simulink model "vardownsampler"  (Simulink 7.3)
settings: Solver=VariableStepDiscrete  StartTime=0.0  StopTime=simTime*SampleTime  RelTol=1e-3
PreLoadFcn:
  | setup_vardownsampler
InitFcn:
  | setup_vardownsampler
values from neighbouring files (symbols this model uses):
  accumOutShift = [1 4 3 2 4]    [setup_vardownsampler.m]    (also in setup_vardownsamplerL8.m = [3 3 2 2 2])
  accumOutWidth = dataWidth + ceil(log2(Rmax))+0    [setup_vardownsampler.m]    (also in setup_vardownsamplerL8.m)
  adderOutShift = 4*ones(1,numRates)    [setup_vardownsampler.m]    (also in setup_vardownsamplerL8.m = 3*ones(1,numRates))
  adderOutWidth = dataWidth + coeffWidth + ceil(log2(L))    [setup_vardownsampler.m]    (also in setup_vardownsamplerL8.m)
  addrWidth = max(1,ceil(log2(Rmax)))    [setup_vardownsampler.m]    (also in setup_vardownsamplerL8.m)
  ChanCount = 16    [setup_vardownsampler.m]    (also in setup_vardownsamplerL8.m = 1)
  ChanCycleCount = ceil(ChanCount/ChanWireCount)    [setup_vardownsampler.m]    (also in setup_vardownsamplerL8.m)
  ChanWireCount = ceil(ChanCount/Period)    [setup_vardownsampler.m]    (also in setup_vardownsamplerL8.m)
  coeffWidth = 16    [setup_vardownsampler.m]    (also in setup_vardownsamplerL8.m)
  dataWidth = 16    [setup_vardownsampler.m]    (also in setup_vardownsamplerL8.m)
  FirAddr = AccumOutScale + 1    (= 4)    [setup_vardownsampler.m]    (also in setup_vardownsamplerL8.m)
  hmatrix = zeros(2*Rmax, L)    [setup_vardownsampler.m]    (also in setup_vardownsamplerL8.m)
  memAddrWidth = max(1,ceil(log2(Nmax)))    [setup_vardownsampler.m]    (also in setup_vardownsamplerL8.m)
  Nmax = Period*Rmax    [setup_vardownsampler.m]    (also in setup_vardownsamplerL8.m)
  Period = floor(ClockRate / SampleRate)    [setup_vardownsampler.m]    (also in setup_vardownsamplerL8.m)
  R = [1 2 5 8 2]    [setup_vardownsampler.m]    (also in setup_vardownsamplerL8.m = [4 5 7 8 9])
  RateWidth = ceil(log2(Rmax))+1    [setup_vardownsampler.m]    (also in setup_vardownsamplerL8.m)
  resetCntWidth = max(1,ceil(log2(Nmax)))    [setup_vardownsampler.m]    (also in setup_vardownsamplerL8.m)
  Rmax = 16    [setup_vardownsampler.m]    (also in setup_vardownsamplerL8.m = 20)
  SampleTime = 1    [setup_vardownsampler.m]    (also in setup_vardownsamplerL8.m)
undefined symbols (not defined in the file or in its folder): AdvDSPBChannelOutDisplay, AdvDSPBDMemDisplay, bank1, bank2, c4, c5, c6, c7, c8, c9, dpoly, dspba_ChannelInVis, dspba_ChannelOutVis, dspba_internal_get_channel_ports, evalAionMaskParam, hmatrix0, hmatrix1, hmatrix2, hmatrix3, latency, primtype, UseDontCare, value
libraries: DSPBAPrim x314, DSPBAModelBus x24, simulink x12, DSPBABase x6
(part 4 of 4)

== system vardownsampler/FilterSystem/coefficients_gen/c2 ==
  addr : Inport
  offset : Inport  Port=2
  Const : DSPBAPrim/Const  primtype=const  nInputs=0  nOutputs=1  omode=Specify via dialog  otype=sfix(coeffWidth)  scale=2^-15  rndmethod=Unbiased  factor=1  satmethod=Symmetric  shift_vec=[0 1 2 -1]  value=0  inPortNames=['+'; '+';]  outPortNames=[' ']  image=dspba_prim.jpg  text=fprintf('%s', num2str(value));  style=Optimised  visibilities=8 + 1024  version=20090407
  Const1 : DSPBAPrim/Const  primtype=const  nInputs=0  nOutputs=1  omode=boolean  otype=sfix(16)  scale=2^-15  rndmethod=Unbiased  factor=1  satmethod=Symmetric  shift_vec=[0 1 2 -1]  value=0  inPortNames=['+'; '+';]  outPortNames=[' ']  image=dspba_prim.jpg  text=fprintf('%s', num2str(value));  style=Optimised  visibilities=8 + 1024  version=20090407
  Const2 : DSPBAPrim/Const  primtype=const  nInputs=0  nOutputs=1  omode=Specify via dialog  otype=sfix(coeffWidth)  scale=2^-15  rndmethod=Unbiased  factor=1  satmethod=Symmetric  shift_vec=[0 1 2 -1]  value=0  inPortNames=['+'; '+';]  outPortNames=[' ']  image=dspba_prim.jpg  text=fprintf('%s', num2str(value));  style=Optimised  visibilities=8 + 1024  version=20090407
  Const3 : DSPBAPrim/Const  primtype=const  nInputs=0  nOutputs=1  omode=boolean  otype=sfix(16)  scale=2^-15  rndmethod=Unbiased  factor=1  satmethod=Symmetric  shift_vec=[0 1 2 -1]  value=0  inPortNames=['+'; '+';]  outPortNames=[' ']  image=dspba_prim.jpg  text=fprintf('%s', num2str(value));  style=Optimised  visibilities=8 + 1024  version=20090407
  LUT0 : DSPBAModelBus/SharedMem  mem_addr=FirAddr+ 4*Rmax  mem_rwmode=Read/Write  mem_data=hmatrix(1:Rmax,3)  mem_init=on  mem_desc=hmatrix2-bank1  mem_type=sfix(coeffWidth)  mem_scale=2^-(coeffWidth-1)  SampleTime=-1  version=20090407
  LUT1 : DSPBAModelBus/SharedMem  mem_addr=FirAddr+ 5*Rmax  mem_rwmode=Read/Write  mem_data=hmatrix(Rmax+1:2*Rmax,3)  mem_init=on  mem_desc=hmatrix2-bank2  mem_type=sfix(coeffWidth)  mem_scale=2^-(coeffWidth-1)  SampleTime=-1  version=20090407
  Mux : DSPBAPrim/Mux  primtype=mux  nInputs=evalAionMaskParam(gcb,'value',1)+1  nOutputs=1  omode=Inherit via internal rule  otype=sfix(16)  scale=2^-15  rndmethod=Unbiased  factor=1  satmethod=Symmetric  shift_vec=[0 1 2 -1]  value=2  inPortNames=['s'; 'd0'; 'd1'; 'd2'; 'd3'; 'd4'; 'd5'; 'd6'; 'd7'; 'd8'; 'd9';]  outPortNames=[' ']  image=dspba_prim.jpg  text=fprintf('%s', primtype);  style=Optimised  visibilities=1032  version=20090623
  Out1 : Outport
  wires:
  addr/1 -> LUT0/1, LUT1/1
  Const2/1 -> LUT1/2
  Const3/1 -> LUT1/3
  Const/1 -> LUT0/2
  Const1/1 -> LUT0/3
  Mux/1 -> Out1/1
  offset/1 -> Mux/1
  LUT0/1 -> Mux/2
  LUT1/1 -> Mux/3

== system vardownsampler/FilterSystem/coefficients_gen/c3 ==
  addr : Inport
  offset : Inport  Port=2
  Const : DSPBAPrim/Const  primtype=const  nInputs=0  nOutputs=1  omode=Specify via dialog  otype=sfix(coeffWidth)  scale=2^-15  rndmethod=Unbiased  factor=1  satmethod=Symmetric  shift_vec=[0 1 2 -1]  value=0  inPortNames=['+'; '+';]  outPortNames=[' ']  image=dspba_prim.jpg  text=fprintf('%s', num2str(value));  style=Optimised  visibilities=8 + 1024  version=20090407
  Const1 : DSPBAPrim/Const  primtype=const  nInputs=0  nOutputs=1  omode=boolean  otype=sfix(16)  scale=2^-15  rndmethod=Unbiased  factor=1  satmethod=Symmetric  shift_vec=[0 1 2 -1]  value=0  inPortNames=['+'; '+';]  outPortNames=[' ']  image=dspba_prim.jpg  text=fprintf('%s', num2str(value));  style=Optimised  visibilities=8 + 1024  version=20090407
  Const2 : DSPBAPrim/Const  primtype=const  nInputs=0  nOutputs=1  omode=Specify via dialog  otype=sfix(coeffWidth)  scale=2^-15  rndmethod=Unbiased  factor=1  satmethod=Symmetric  shift_vec=[0 1 2 -1]  value=0  inPortNames=['+'; '+';]  outPortNames=[' ']  image=dspba_prim.jpg  text=fprintf('%s', num2str(value));  style=Optimised  visibilities=8 + 1024  version=20090407
  Const3 : DSPBAPrim/Const  primtype=const  nInputs=0  nOutputs=1  omode=boolean  otype=sfix(16)  scale=2^-15  rndmethod=Unbiased  factor=1  satmethod=Symmetric  shift_vec=[0 1 2 -1]  value=0  inPortNames=['+'; '+';]  outPortNames=[' ']  image=dspba_prim.jpg  text=fprintf('%s', num2str(value));  style=Optimised  visibilities=8 + 1024  version=20090407
  LUT1 : DSPBAModelBus/SharedMem  mem_addr=FirAddr+ 7*Rmax  mem_rwmode=Read/Write  mem_data=hmatrix(Rmax+1:2*Rmax,4)  mem_init=on  mem_desc=hmatrix3-bank2  mem_type=sfix(coeffWidth)  mem_scale=2^-(coeffWidth-1)  SampleTime=-1  version=20090407
  LUT3 : DSPBAModelBus/SharedMem  mem_addr=FirAddr+ 6*Rmax  mem_rwmode=Read/Write  mem_data=hmatrix(1:Rmax,4)  mem_init=on  mem_desc=hmatrix3-bank1  mem_type=sfix(coeffWidth)  mem_scale=2^-(coeffWidth-1)  SampleTime=-1  version=20090407
  Mux : DSPBAPrim/Mux  primtype=mux  nInputs=evalAionMaskParam(gcb,'value',1)+1  nOutputs=1  omode=Inherit via internal rule  otype=sfix(16)  scale=2^-15  rndmethod=Unbiased  factor=1  satmethod=Symmetric  shift_vec=[0 1 2 -1]  value=2  inPortNames=['s'; 'd0'; 'd1'; 'd2'; 'd3'; 'd4'; 'd5'; 'd6'; 'd7'; 'd8'; 'd9';]  outPortNames=[' ']  image=dspba_prim.jpg  text=fprintf('%s', primtype);  style=Optimised  visibilities=1032  version=20090623
  c3 : Outport
  wires:
  addr/1 -> LUT3/1, LUT1/1
  Const/1 -> LUT3/2
  Const1/1 -> LUT3/3
  Const2/1 -> LUT1/2
  Const3/1 -> LUT1/3
  offset/1 -> Mux/1
  LUT3/1 -> Mux/2
  LUT1/1 -> Mux/3
  Mux/1 -> c3/1

== system vardownsampler/FilterSystem/coefficients_gen/c4 ==
  addr : Inport
  offset : Inport  Port=2
  Const : DSPBAPrim/Const  primtype=const  nInputs=0  nOutputs=1  omode=Specify via dialog  otype=sfix(coeffWidth)  scale=2^-15  rndmethod=Unbiased  factor=1  satmethod=Symmetric  shift_vec=[0 1 2 -1]  value=0  inPortNames=['+'; '+';]  outPortNames=[' ']  image=dspba_prim.jpg  text=fprintf('%s', num2str(value));  style=Optimised  visibilities=8 + 1024  version=20090407
  Const1 : DSPBAPrim/Const  primtype=const  nInputs=0  nOutputs=1  omode=boolean  otype=sfix(16)  scale=2^-15  rndmethod=Unbiased  factor=1  satmethod=Symmetric  shift_vec=[0 1 2 -1]  value=0  inPortNames=['+'; '+';]  outPortNames=[' ']  image=dspba_prim.jpg  text=fprintf('%s', num2str(value));  style=Optimised  visibilities=8 + 1024  version=20090407
  Const2 : DSPBAPrim/Const  primtype=const  nInputs=0  nOutputs=1  omode=Specify via dialog  otype=sfix(coeffWidth)  scale=2^-15  rndmethod=Unbiased  factor=1  satmethod=Symmetric  shift_vec=[0 1 2 -1]  value=0  inPortNames=['+'; '+';]  outPortNames=[' ']  image=dspba_prim.jpg  text=fprintf('%s', num2str(value));  style=Optimised  visibilities=8 + 1024  version=20090407
  Const3 : DSPBAPrim/Const  primtype=const  nInputs=0  nOutputs=1  omode=boolean  otype=sfix(16)  scale=2^-15  rndmethod=Unbiased  factor=1  satmethod=Symmetric  shift_vec=[0 1 2 -1]  value=0  inPortNames=['+'; '+';]  outPortNames=[' ']  image=dspba_prim.jpg  text=fprintf('%s', num2str(value));  style=Optimised  visibilities=8 + 1024  version=20090407
  LUT0 : DSPBAModelBus/SharedMem  mem_addr=FirAddr+8*Rmax  mem_rwmode=Read/Write  mem_data=hmatrix(1:Rmax,5)  mem_init=on  mem_desc=c4-bank1  mem_type=sfix(coeffWidth)  mem_scale=2^-(coeffWidth-1)  SampleTime=-1  version=20090407
  LUT1 : DSPBAModelBus/SharedMem  mem_addr=FirAddr+9*Rmax  mem_rwmode=Read/Write  mem_data=hmatrix(Rmax+1:2*Rmax,5)  mem_init=on  mem_desc=c4-bank2  mem_type=sfix(coeffWidth)  mem_scale=2^-(coeffWidth-1)  SampleTime=-1  version=20090407
  Mux : DSPBAPrim/Mux  primtype=mux  nInputs=evalAionMaskParam(gcb,'value',1)+1  nOutputs=1  omode=Inherit via internal rule  otype=sfix(16)  scale=2^-15  rndmethod=Unbiased  factor=1  satmethod=Symmetric  shift_vec=[0 1 2 -1]  value=2  inPortNames=['s'; 'd0'; 'd1'; 'd2'; 'd3'; 'd4'; 'd5'; 'd6'; 'd7'; 'd8'; 'd9';]  outPortNames=[' ']  image=dspba_prim.jpg  text=fprintf('%s', primtype);  style=Optimised  visibilities=1032  version=20090623
  c4 : Outport
  wires:
  addr/1 -> LUT0/1, LUT1/1
  Const/1 -> LUT0/2
  Const1/1 -> LUT0/3
  Const2/1 -> LUT1/2
  Const3/1 -> LUT1/3
  offset/1 -> Mux/1
  LUT0/1 -> Mux/2
  LUT1/1 -> Mux/3
  Mux/1 -> c4/1

== system vardownsampler/FilterSystem/coefficients_gen/c5 ==
  addr : Inport
  offset : Inport  Port=2
  Const : DSPBAPrim/Const  primtype=const  nInputs=0  nOutputs=1  omode=Specify via dialog  otype=sfix(coeffWidth)  scale=2^-15  rndmethod=Unbiased  factor=1  satmethod=Symmetric  shift_vec=[0 1 2 -1]  value=0  inPortNames=['+'; '+';]  outPortNames=[' ']  image=dspba_prim.jpg  text=fprintf('%s', num2str(value));  style=Optimised  visibilities=8 + 1024  version=20090407
  Const1 : DSPBAPrim/Const  primtype=const  nInputs=0  nOutputs=1  omode=boolean  otype=sfix(16)  scale=2^-15  rndmethod=Unbiased  factor=1  satmethod=Symmetric  shift_vec=[0 1 2 -1]  value=0  inPortNames=['+'; '+';]  outPortNames=[' ']  image=dspba_prim.jpg  text=fprintf('%s', num2str(value));  style=Optimised  visibilities=8 + 1024  version=20090407
  Const2 : DSPBAPrim/Const  primtype=const  nInputs=0  nOutputs=1  omode=Specify via dialog  otype=sfix(coeffWidth)  scale=2^-15  rndmethod=Unbiased  factor=1  satmethod=Symmetric  shift_vec=[0 1 2 -1]  value=0  inPortNames=['+'; '+';]  outPortNames=[' ']  image=dspba_prim.jpg  text=fprintf('%s', num2str(value));  style=Optimised  visibilities=8 + 1024  version=20090407
  Const3 : DSPBAPrim/Const  primtype=const  nInputs=0  nOutputs=1  omode=boolean  otype=sfix(16)  scale=2^-15  rndmethod=Unbiased  factor=1  satmethod=Symmetric  shift_vec=[0 1 2 -1]  value=0  inPortNames=['+'; '+';]  outPortNames=[' ']  image=dspba_prim.jpg  text=fprintf('%s', num2str(value));  style=Optimised  visibilities=8 + 1024  version=20090407
  LUT1 : DSPBAModelBus/SharedMem  mem_addr=FirAddr+11*Rmax  mem_rwmode=Read/Write  mem_data=hmatrix(Rmax+1:2*Rmax,6)  mem_init=on  mem_desc=c5-bank2  mem_type=sfix(coeffWidth)  mem_scale=2^-(coeffWidth-1)  SampleTime=-1  version=20090407
  LUT5 : DSPBAModelBus/SharedMem  mem_addr=FirAddr+10*Rmax  mem_rwmode=Read/Write  mem_data=hmatrix(1:Rmax,6)  mem_init=on  mem_desc=c5-bank1  mem_type=sfix(coeffWidth)  mem_scale=2^-(coeffWidth-1)  SampleTime=-1  version=20090407
  Mux : DSPBAPrim/Mux  primtype=mux  nInputs=evalAionMaskParam(gcb,'value',1)+1  nOutputs=1  omode=Inherit via internal rule  otype=sfix(16)  scale=2^-15  rndmethod=Unbiased  factor=1  satmethod=Symmetric  shift_vec=[0 1 2 -1]  value=2  inPortNames=['s'; 'd0'; 'd1'; 'd2'; 'd3'; 'd4'; 'd5'; 'd6'; 'd7'; 'd8'; 'd9';]  outPortNames=[' ']  image=dspba_prim.jpg  text=fprintf('%s', primtype);  style=Optimised  visibilities=1032  version=20090623
  c3 : Outport
  wires:
  addr/1 -> LUT5/1, LUT1/1
  Const/1 -> LUT5/2
  Const1/1 -> LUT5/3
  Const2/1 -> LUT1/2
  Const3/1 -> LUT1/3
  offset/1 -> Mux/1
  LUT5/1 -> Mux/2
  LUT1/1 -> Mux/3
  Mux/1 -> c3/1

== system vardownsampler/FilterSystem/coefficients_gen/c6 ==
  addr : Inport
  offset : Inport  Port=2
  Const : DSPBAPrim/Const  primtype=const  nInputs=0  nOutputs=1  omode=Specify via dialog  otype=sfix(coeffWidth)  scale=2^-15  rndmethod=Unbiased  factor=1  satmethod=Symmetric  shift_vec=[0 1 2 -1]  value=0  inPortNames=['+'; '+';]  outPortNames=[' ']  image=dspba_prim.jpg  text=fprintf('%s', num2str(value));  style=Optimised  visibilities=8 + 1024  version=20090407
  Const1 : DSPBAPrim/Const  primtype=const  nInputs=0  nOutputs=1  omode=boolean  otype=sfix(16)  scale=2^-15  rndmethod=Unbiased  factor=1  satmethod=Symmetric  shift_vec=[0 1 2 -1]  value=0  inPortNames=['+'; '+';]  outPortNames=[' ']  image=dspba_prim.jpg  text=fprintf('%s', num2str(value));  style=Optimised  visibilities=8 + 1024  version=20090407
  Const2 : DSPBAPrim/Const  primtype=const  nInputs=0  nOutputs=1  omode=Specify via dialog  otype=sfix(coeffWidth)  scale=2^-15  rndmethod=Unbiased  factor=1  satmethod=Symmetric  shift_vec=[0 1 2 -1]  value=0  inPortNames=['+'; '+';]  outPortNames=[' ']  image=dspba_prim.jpg  text=fprintf('%s', num2str(value));  style=Optimised  visibilities=8 + 1024  version=20090407
  Const3 : DSPBAPrim/Const  primtype=const  nInputs=0  nOutputs=1  omode=boolean  otype=sfix(16)  scale=2^-15  rndmethod=Unbiased  factor=1  satmethod=Symmetric  shift_vec=[0 1 2 -1]  value=0  inPortNames=['+'; '+';]  outPortNames=[' ']  image=dspba_prim.jpg  text=fprintf('%s', num2str(value));  style=Optimised  visibilities=8 + 1024  version=20090407
  LUT0 : DSPBAModelBus/SharedMem  mem_addr=FirAddr+12*Rmax  mem_rwmode=Read/Write  mem_data=hmatrix(1:Rmax,7)  mem_init=on  mem_desc=c6-bank1  mem_type=sfix(coeffWidth)  mem_scale=2^-(coeffWidth-1)  SampleTime=-1  version=20090407
  LUT1 : DSPBAModelBus/SharedMem  mem_addr=FirAddr+13*Rmax  mem_rwmode=Read/Write  mem_data=hmatrix(Rmax+1:2*Rmax,7)  mem_init=on  mem_desc=c6-bank2  mem_type=sfix(coeffWidth)  mem_scale=2^-(coeffWidth-1)  SampleTime=-1  version=20090407
  Mux : DSPBAPrim/Mux  primtype=mux  nInputs=evalAionMaskParam(gcb,'value',1)+1  nOutputs=1  omode=Inherit via internal rule  otype=sfix(16)  scale=2^-15  rndmethod=Unbiased  factor=1  satmethod=Symmetric  shift_vec=[0 1 2 -1]  value=2  inPortNames=['s'; 'd0'; 'd1'; 'd2'; 'd3'; 'd4'; 'd5'; 'd6'; 'd7'; 'd8'; 'd9';]  outPortNames=[' ']  image=dspba_prim.jpg  text=fprintf('%s', primtype);  style=Optimised  visibilities=1032  version=20090623
  c6 : Outport
  wires:
  addr/1 -> LUT0/1, LUT1/1
  Const/1 -> LUT0/2
  Const1/1 -> LUT0/3
  Const2/1 -> LUT1/2
  Const3/1 -> LUT1/3
  offset/1 -> Mux/1
  LUT0/1 -> Mux/2
  LUT1/1 -> Mux/3
  Mux/1 -> c6/1

== system vardownsampler/FilterSystem/coefficients_gen/c7 ==
  addr : Inport
  offset : Inport  Port=2
  Const : DSPBAPrim/Const  primtype=const  nInputs=0  nOutputs=1  omode=Specify via dialog  otype=sfix(coeffWidth)  scale=2^-15  rndmethod=Unbiased  factor=1  satmethod=Symmetric  shift_vec=[0 1 2 -1]  value=0  inPortNames=['+'; '+';]  outPortNames=[' ']  image=dspba_prim.jpg  text=fprintf('%s', num2str(value));  style=Optimised  visibilities=8 + 1024  version=20090407
  Const1 : DSPBAPrim/Const  primtype=const  nInputs=0  nOutputs=1  omode=boolean  otype=sfix(16)  scale=2^-15  rndmethod=Unbiased  factor=1  satmethod=Symmetric  shift_vec=[0 1 2 -1]  value=0  inPortNames=['+'; '+';]  outPortNames=[' ']  image=dspba_prim.jpg  text=fprintf('%s', num2str(value));  style=Optimised  visibilities=8 + 1024  version=20090407
  Const2 : DSPBAPrim/Const  primtype=const  nInputs=0  nOutputs=1  omode=Specify via dialog  otype=sfix(coeffWidth)  scale=2^-15  rndmethod=Unbiased  factor=1  satmethod=Symmetric  shift_vec=[0 1 2 -1]  value=0  inPortNames=['+'; '+';]  outPortNames=[' ']  image=dspba_prim.jpg  text=fprintf('%s', num2str(value));  style=Optimised  visibilities=8 + 1024  version=20090407
  Const3 : DSPBAPrim/Const  primtype=const  nInputs=0  nOutputs=1  omode=boolean  otype=sfix(16)  scale=2^-15  rndmethod=Unbiased  factor=1  satmethod=Symmetric  shift_vec=[0 1 2 -1]  value=0  inPortNames=['+'; '+';]  outPortNames=[' ']  image=dspba_prim.jpg  text=fprintf('%s', num2str(value));  style=Optimised  visibilities=8 + 1024  version=20090407
  LUT1 : DSPBAModelBus/SharedMem  mem_addr=FirAddr+15*Rmax  mem_rwmode=Read/Write  mem_data=hmatrix(Rmax+1:2*Rmax,8)  mem_init=on  mem_desc=c7-bank2  mem_type=sfix(coeffWidth)  mem_scale=2^-(coeffWidth-1)  SampleTime=-1  version=20090407
  LUT7 : DSPBAModelBus/SharedMem  mem_addr=FirAddr+14*Rmax  mem_rwmode=Read/Write  mem_data=hmatrix(1:Rmax,8)  mem_init=on  mem_desc=c7-bank1  mem_type=sfix(coeffWidth)  mem_scale=2^-(coeffWidth-1)  SampleTime=-1  version=20090407
  Mux : DSPBAPrim/Mux  primtype=mux  nInputs=evalAionMaskParam(gcb,'value',1)+1  nOutputs=1  omode=Inherit via internal rule  otype=sfix(16)  scale=2^-15  rndmethod=Unbiased  factor=1  satmethod=Symmetric  shift_vec=[0 1 2 -1]  value=2  inPortNames=['s'; 'd0'; 'd1'; 'd2'; 'd3'; 'd4'; 'd5'; 'd6'; 'd7'; 'd8'; 'd9';]  outPortNames=[' ']  image=dspba_prim.jpg  text=fprintf('%s', primtype);  style=Optimised  visibilities=1032  version=20090623
  c7 : Outport
  wires:
  addr/1 -> LUT7/1, LUT1/1
  Const/1 -> LUT7/2
  Const1/1 -> LUT7/3
  Const2/1 -> LUT1/2
  Const3/1 -> LUT1/3
  offset/1 -> Mux/1
  LUT7/1 -> Mux/2
  LUT1/1 -> Mux/3
  Mux/1 -> c7/1

== system vardownsampler/FilterSystem/coefficients_gen/c8 ==
  addr : Inport
  offset : Inport  Port=2
  Const : DSPBAPrim/Const  primtype=const  nInputs=0  nOutputs=1  omode=Specify via dialog  otype=sfix(coeffWidth)  scale=2^-15  rndmethod=Unbiased  factor=1  satmethod=Symmetric  shift_vec=[0 1 2 -1]  value=0  inPortNames=['+'; '+';]  outPortNames=[' ']  image=dspba_prim.jpg  text=fprintf('%s', num2str(value));  style=Optimised  visibilities=8 + 1024  version=20090407
  Const1 : DSPBAPrim/Const  primtype=const  nInputs=0  nOutputs=1  omode=boolean  otype=sfix(16)  scale=2^-15  rndmethod=Unbiased  factor=1  satmethod=Symmetric  shift_vec=[0 1 2 -1]  value=0  inPortNames=['+'; '+';]  outPortNames=[' ']  image=dspba_prim.jpg  text=fprintf('%s', num2str(value));  style=Optimised  visibilities=8 + 1024  version=20090407
  Const2 : DSPBAPrim/Const  primtype=const  nInputs=0  nOutputs=1  omode=Specify via dialog  otype=sfix(coeffWidth)  scale=2^-15  rndmethod=Unbiased  factor=1  satmethod=Symmetric  shift_vec=[0 1 2 -1]  value=0  inPortNames=['+'; '+';]  outPortNames=[' ']  image=dspba_prim.jpg  text=fprintf('%s', num2str(value));  style=Optimised  visibilities=8 + 1024  version=20090407
  Const3 : DSPBAPrim/Const  primtype=const  nInputs=0  nOutputs=1  omode=boolean  otype=sfix(16)  scale=2^-15  rndmethod=Unbiased  factor=1  satmethod=Symmetric  shift_vec=[0 1 2 -1]  value=0  inPortNames=['+'; '+';]  outPortNames=[' ']  image=dspba_prim.jpg  text=fprintf('%s', num2str(value));  style=Optimised  visibilities=8 + 1024  version=20090407
  LUT1 : DSPBAModelBus/SharedMem  mem_addr=FirAddr+17*Rmax  mem_rwmode=Read/Write  mem_data=hmatrix(Rmax+1:2*Rmax,9)  mem_init=on  mem_desc=c8-bank2  mem_type=sfix(coeffWidth)  mem_scale=2^-(coeffWidth-1)  SampleTime=-1  version=20090407
  LUT8 : DSPBAModelBus/SharedMem  mem_addr=FirAddr+16*Rmax  mem_rwmode=Read/Write  mem_data=hmatrix(1:Rmax,9)  mem_init=on  mem_desc=c8-bank1  mem_type=sfix(coeffWidth)  mem_scale=2^-(coeffWidth-1)  SampleTime=-1  version=20090407
  Mux : DSPBAPrim/Mux  primtype=mux  nInputs=evalAionMaskParam(gcb,'value',1)+1  nOutputs=1  omode=Inherit via internal rule  otype=sfix(16)  scale=2^-15  rndmethod=Unbiased  factor=1  satmethod=Symmetric  shift_vec=[0 1 2 -1]  value=2  inPortNames=['s'; 'd0'; 'd1'; 'd2'; 'd3'; 'd4'; 'd5'; 'd6'; 'd7'; 'd8'; 'd9';]  outPortNames=[' ']  image=dspba_prim.jpg  text=fprintf('%s', primtype);  style=Optimised  visibilities=1032  version=20090623
  c8 : Outport
  wires:
  addr/1 -> LUT8/1, LUT1/1
  Const/1 -> LUT8/2
  Const1/1 -> LUT8/3
  Const2/1 -> LUT1/2
  Const3/1 -> LUT1/3
  offset/1 -> Mux/1
  LUT8/1 -> Mux/2
  LUT1/1 -> Mux/3
  Mux/1 -> c8/1

== system vardownsampler/FilterSystem/coefficients_gen/c9 ==
  addr : Inport
  offset : Inport  Port=2
  Const : DSPBAPrim/Const  primtype=const  nInputs=0  nOutputs=1  omode=Specify via dialog  otype=sfix(coeffWidth)  scale=2^-15  rndmethod=Unbiased  factor=1  satmethod=Symmetric  shift_vec=[0 1 2 -1]  value=0  inPortNames=['+'; '+';]  outPortNames=[' ']  image=dspba_prim.jpg  text=fprintf('%s', num2str(value));  style=Optimised  visibilities=8 + 1024  version=20090407
  Const1 : DSPBAPrim/Const  primtype=const  nInputs=0  nOutputs=1  omode=boolean  otype=sfix(16)  scale=2^-15  rndmethod=Unbiased  factor=1  satmethod=Symmetric  shift_vec=[0 1 2 -1]  value=0  inPortNames=['+'; '+';]  outPortNames=[' ']  image=dspba_prim.jpg  text=fprintf('%s', num2str(value));  style=Optimised  visibilities=8 + 1024  version=20090407
  Const2 : DSPBAPrim/Const  primtype=const  nInputs=0  nOutputs=1  omode=Specify via dialog  otype=sfix(coeffWidth)  scale=2^-15  rndmethod=Unbiased  factor=1  satmethod=Symmetric  shift_vec=[0 1 2 -1]  value=0  inPortNames=['+'; '+';]  outPortNames=[' ']  image=dspba_prim.jpg  text=fprintf('%s', num2str(value));  style=Optimised  visibilities=8 + 1024  version=20090407
  Const3 : DSPBAPrim/Const  primtype=const  nInputs=0  nOutputs=1  omode=boolean  otype=sfix(16)  scale=2^-15  rndmethod=Unbiased  factor=1  satmethod=Symmetric  shift_vec=[0 1 2 -1]  value=0  inPortNames=['+'; '+';]  outPortNames=[' ']  image=dspba_prim.jpg  text=fprintf('%s', num2str(value));  style=Optimised  visibilities=8 + 1024  version=20090407
  LUT1 : DSPBAModelBus/SharedMem  mem_addr=FirAddr+19*Rmax  mem_rwmode=Read/Write  mem_data=hmatrix(Rmax+1:2*Rmax,10)  mem_init=on  mem_desc=c9-bank2  mem_type=sfix(coeffWidth)  mem_scale=2^-(coeffWidth-1)  SampleTime=-1  version=20090407
  LUT9 : DSPBAModelBus/SharedMem  mem_addr=FirAddr+18*Rmax  mem_rwmode=Read/Write  mem_data=hmatrix(1:Rmax,10)  mem_init=on  mem_desc=c9-bank1  mem_type=sfix(coeffWidth)  mem_scale=2^-(coeffWidth-1)  SampleTime=-1  version=20090407
  Mux : DSPBAPrim/Mux  primtype=mux  nInputs=evalAionMaskParam(gcb,'value',1)+1  nOutputs=1  omode=Inherit via internal rule  otype=sfix(16)  scale=2^-15  rndmethod=Unbiased  factor=1  satmethod=Symmetric  shift_vec=[0 1 2 -1]  value=2  inPortNames=['s'; 'd0'; 'd1'; 'd2'; 'd3'; 'd4'; 'd5'; 'd6'; 'd7'; 'd8'; 'd9';]  outPortNames=[' ']  image=dspba_prim.jpg  text=fprintf('%s', primtype);  style=Optimised  visibilities=1032  version=20090623
  c9 : Outport
  wires:
  addr/1 -> LUT9/1, LUT1/1
  Const/1 -> LUT9/2
  Const1/1 -> LUT9/3
  Const2/1 -> LUT1/2
  Const3/1 -> LUT1/3
  offset/1 -> Mux/1
  LUT9/1 -> Mux/2
  LUT1/1 -> Mux/3
  Mux/1 -> c9/1

== system vardownsampler/FilterSystem/gen_addr_control/coeff_cnt ==
  note: s=0, no rate transition
  rate : Inport
  transig : Inport  Port=2
  AddSLoad : DSPBAPrim/AddSLoad  primtype=addsload  nInputs=4  nOutputs=1  omode=Specify via dialog  otype=uint(addrWidth)  scale=1  rndmethod=Unbiased  factor=1  satmethod=Symmetric  shift_vec=[0 1 2 -1]  value=0  inPortNames=['+'; '+'; 's'; 'v']  outPortNames=[' ']  image=dspba_prim.jpg  text=fprintf('+');  style=Optimised  visibilities=8  version=20090407
  CmpEQ : DSPBAPrim/CmpEQ  primtype=cmpeq  nInputs=2  nOutputs=1  omode=boolean  otype=sfix(16)  scale=2^-15  rndmethod=Unbiased  factor=1  satmethod=Symmetric  shift_vec=[0 1 2 -1]  value=0  inPortNames=[' '; ' ';]  outPortNames=[' ']  image=dspba_prim.jpg  text=fprintf('==');  style=Optimised  visibilities=0  version=20090407
  Const1 : DSPBAPrim/Const  primtype=const  nInputs=0  nOutputs=1  omode=Specify via dialog  otype=uint(addrWidth)  scale=1  rndmethod=Unbiased  factor=1  satmethod=Symmetric  shift_vec=[0 1 2 -1]  value=1  inPortNames=['+'; '+';]  outPortNames=[' ']  image=dspba_prim.jpg  text=fprintf('%s', num2str(value));  style=Optimised  visibilities=8 + 1024  version=20090407
  Const2 : DSPBAPrim/Const  primtype=const  nInputs=0  nOutputs=1  omode=Specify via dialog  otype=uint(addrWidth)  scale=1  rndmethod=Unbiased  factor=1  satmethod=Symmetric  shift_vec=[0 1 2 -1]  value=1  inPortNames=['+'; '+';]  outPortNames=[' ']  image=dspba_prim.jpg  text=fprintf('%s', num2str(value));  style=Optimised  visibilities=8 + 1024  version=20090407
  Const3 : DSPBAPrim/Const  primtype=const  nInputs=0  nOutputs=1  omode=Specify via dialog  otype=uint(addrWidth)  scale=1  rndmethod=Unbiased  factor=1  satmethod=Symmetric  shift_vec=[0 1 2 -1]  value=0  inPortNames=['+'; '+';]  outPortNames=[' ']  image=dspba_prim.jpg  text=fprintf('%s', num2str(value));  style=Optimised  visibilities=8 + 1024  version=20090407
  Mux : DSPBAPrim/Mux  primtype=mux  nInputs=evalAionMaskParam(gcb,'value',1)+1  nOutputs=1  omode=Inherit via internal rule  otype=sfix(16)  scale=2^-15  rndmethod=Unbiased  factor=1  satmethod=Symmetric  shift_vec=[0 1 2 -1]  value=2  inPortNames=['s'; 'd0'; 'd1'; 'd2'; 'd3'; 'd4'; 'd5'; 'd6'; 'd7'; 'd8'; 'd9';]  outPortNames=[' ']  image=dspba_prim.jpg  text=fprintf('%s', primtype);  style=Optimised  visibilities=1032  version=20090623
  Not : DSPBAPrim/Not  primtype=not  nInputs=1  nOutputs=1  omode=Inherit via internal rule  otype=sfix(16)  scale=2^-15  rndmethod=Unbiased  factor=1  satmethod=Symmetric  shift_vec=[0 1 2 -1]  value=0  inPortNames=[' '; ' ';]  outPortNames=[' ']  image=dspba_prim.jpg  text=fprintf('~');  style=Optimised  visibilities=8  version=20090407
  Or : DSPBAPrim/Or  primtype=or  nInputs=2  nOutputs=1  omode=Inherit via internal rule  otype=sfix(16)  scale=2^-15  rndmethod=Unbiased  factor=1  satmethod=Symmetric  shift_vec=[0 1 2 -1]  value=0  inPortNames=[' '; ' '; ' '; ' '; ' '; ' '; ' '; ' '; ' '; ' '; ' '; ' '; ' '; ' '; ' '; ' '; ]  outPortNames=[' ']  image=dspba_prim.jpg  text=fprintf('|');  style=Optimised  visibilities=8+2  version=20090407
  SampleDelay : DSPBAPrim/SampleDelay  primtype=sampdelay  nInputs=1  nOutputs=1  omode=Specify via dialog  otype=uint(addrWidth)  scale=1  rndmethod=Unbiased  factor=1  satmethod=Symmetric  shift_vec=[0 1 2 -1]  value=Period  inPortNames=[' '; ' ';]  outPortNames=[' ']  image=dspba_prim.jpg  text=dpoly(1, eye(1,value+1), 'z')  style=Optimised  visibilities=8 + 1024  version=20090407
  SampleDelay1 : DSPBAPrim/SampleDelay  primtype=sampdelay  nInputs=1  nOutputs=1  omode=boolean  otype=sfix(16)  scale=2^-15  rndmethod=Unbiased  factor=1  satmethod=Symmetric  shift_vec=[0 1 2 -1]  value=1  inPortNames=[' '; ' ';]  outPortNames=[' ']  image=dspba_prim.jpg  text=dpoly(1, eye(1,value+1), 'z')  style=Optimised  visibilities=8 + 1024  version=20090407
  SampleDelay2 : DSPBAPrim/SampleDelay  primtype=sampdelay  nInputs=1  nOutputs=1  omode=boolean  otype=sfix(16)  scale=2^-15  rndmethod=Unbiased  factor=1  satmethod=Symmetric  shift_vec=[0 1 2 -1]  value=Period  inPortNames=[' '; ' ';]  outPortNames=[' ']  image=dspba_prim.jpg  text=dpoly(1, eye(1,value+1), 'z')  style=Optimised  visibilities=8 + 1024  version=20090407
  Sub : DSPBAPrim/Sub  primtype=sub  nInputs=2  nOutputs=1  omode=Specify via dialog  otype=uint(addrWidth)  scale=1  rndmethod=Unbiased  factor=1  satmethod=Symmetric  shift_vec=[0 1 2 -1]  value=0  inPortNames=['+'; '-';]  outPortNames=[' ']  image=dspba_prim.jpg  text=fprintf('-');  style=Optimised  visibilities=8  version=20090407
  Xor : DSPBAPrim/Xor  primtype=xor  nInputs=2  nOutputs=1  omode=Inherit via internal rule  otype=sfix(16)  scale=2^-15  rndmethod=Unbiased  factor=1  satmethod=Symmetric  shift_vec=[0 1 2 -1]  value=0  inPortNames=[' '; ' '; ' '; ' '; ' '; ' '; ' '; ' '; ' '; ' '; ' '; ' '; ' '; ' '; ' '; ' '; ]  outPortNames=[' ']  image=dspba_prim.jpg  text=fprintf('^');  style=Optimised  visibilities=8+2  version=20090407
  coeff_cnt : Outport
  wires:
  Const1/1 -> AddSLoad/2
  AddSLoad/1 -> SampleDelay/1, coeff_cnt/1
  SampleDelay/1 -> AddSLoad/1, CmpEQ/1  "cnt"
  Const2/1 -> Sub/2
  Sub/1 -> CmpEQ/2
  Const3/1 -> AddSLoad/4
  rate/1 -> Sub/1
  CmpEQ/1 -> Or/1
  transig/1 -> SampleDelay2/1, Xor/2
  Or/1 -> AddSLoad/3
  Not/1 -> Mux/3
  SampleDelay1/1 -> Not/1, Mux/2  "flag_n_1"
  Mux/1 -> SampleDelay1/1, Or/2  "flag_n"
  SampleDelay2/1 -> Xor/1
  Xor/1 -> Mux/1

== system vardownsampler/FilterSystem/gen_addr_control/gen_coeff_offset ==
  note: s=0, no rate transition
  note: Two memory banks are used to store memory coefficients. Each bank has depth Rmax. So the offset is 0 or Rmax.
  transig : Inport
  Const : DSPBAPrim/Const  primtype=const  nInputs=0  nOutputs=1  omode=boolean  otype=ufix(1)  scale=1  rndmethod=Unbiased  factor=1  satmethod=Symmetric  shift_vec=[0 1 2 -1]  value=1  inPortNames=['+'; '+';]  outPortNames=[' ']  image=dspba_prim.jpg  text=fprintf('%s', num2str(value));  style=Optimised  visibilities=8 + 1024  version=20090407
  Const1 : DSPBAPrim/Const  primtype=const  nInputs=0  nOutputs=1  omode=boolean  otype=ufix(1)  scale=1  rndmethod=Unbiased  factor=1  satmethod=Symmetric  shift_vec=[0 1 2 -1]  value=0  inPortNames=['+'; '+';]  outPortNames=[' ']  image=dspba_prim.jpg  text=fprintf('%s', num2str(value));  style=Optimised  visibilities=8 + 1024  version=20090407
  Mux : DSPBAPrim/Mux  primtype=mux  nInputs=evalAionMaskParam(gcb,'value',1)+1  nOutputs=1  omode=Inherit via internal rule  otype=sfix(16)  scale=2^-15  rndmethod=Unbiased  factor=1  satmethod=Symmetric  shift_vec=[0 1 2 -1]  value=2  inPortNames=['s'; 'd0'; 'd1'; 'd2'; 'd3'; 'd4'; 'd5'; 'd6'; 'd7'; 'd8'; 'd9';]  outPortNames=[' ']  image=dspba_prim.jpg  text=fprintf('%s', primtype);  style=Optimised  visibilities=1032  version=20090623
  Mux1 : DSPBAPrim/Mux  primtype=mux  nInputs=evalAionMaskParam(gcb,'value',1)+1  nOutputs=1  omode=Inherit via internal rule  otype=sfix(16)  scale=2^-15  rndmethod=Unbiased  factor=1  satmethod=Symmetric  shift_vec=[0 1 2 -1]  value=2  inPortNames=['s'; 'd0'; 'd1'; 'd2'; 'd3'; 'd4'; 'd5'; 'd6'; 'd7'; 'd8'; 'd9';]  outPortNames=[' ']  image=dspba_prim.jpg  text=fprintf('%s', primtype);  style=Optimised  visibilities=1032  version=20090623
  Not : DSPBAPrim/Not  primtype=not  nInputs=1  nOutputs=1  omode=Inherit via internal rule  otype=sfix(16)  scale=2^-15  rndmethod=Unbiased  factor=1  satmethod=Symmetric  shift_vec=[0 1 2 -1]  value=0  inPortNames=[' '; ' ';]  outPortNames=[' ']  image=dspba_prim.jpg  text=fprintf('~');  style=Optimised  visibilities=8  version=20090407
  SampleDelay1 : DSPBAPrim/SampleDelay  primtype=sampdelay  nInputs=1  nOutputs=1  omode=boolean  otype=sfix(16)  scale=2^-15  rndmethod=Unbiased  factor=1  satmethod=Symmetric  shift_vec=[0 1 2 -1]  value=1  inPortNames=[' '; ' ';]  outPortNames=[' ']  image=dspba_prim.jpg  text=dpoly(1, eye(1,value+1), 'z')  style=Optimised  visibilities=8 + 1024  version=20090407
  coffset : Outport
  wires:
  Not/1 -> Mux/3
  SampleDelay1/1 -> Mux/2, Not/1  "flag_n_1"
  transig/1 -> Mux/1
  Mux/1 -> SampleDelay1/1, Mux1/1  "flag_n"
  Const/1 -> Mux1/2
  Const1/1 -> Mux1/3
  Mux1/1 -> coffset/1

== system vardownsampler/FilterSystem/gen_addr_control/gen_outvalid ==
  in_valid : Inport
  coeff_cnt : Inport  Port=2  OutDataType=fixdt(1, 16)  OutScaling=2^0
  CmpNE : DSPBAPrim/CmpNE  primtype=cmpne  nInputs=2  nOutputs=1  omode=boolean  otype=sfix(16)  scale=2^-15  rndmethod=Unbiased  factor=1  satmethod=Symmetric  shift_vec=[0 1 2 -1]  value=0  inPortNames=[' '; ' ';]  outPortNames=[' ']  image=dspba_prim.jpg  text=fprintf('~=');  style=Optimised  visibilities=0  version=20090407
  Const8 : DSPBAPrim/Const  primtype=const  nInputs=0  nOutputs=1  omode=Specify via dialog  otype=uint(addrWidth)  scale=1  rndmethod=Unbiased  factor=1  satmethod=Symmetric  shift_vec=[0 1 2 -1]  value=0  inPortNames=['+'; '+';]  outPortNames=[' ']  image=dspba_prim.jpg  text=fprintf('%s', num2str(value));  style=Optimised  visibilities=8 + 1024  version=20090407
  Const9 : DSPBAPrim/Const  primtype=const  nInputs=0  nOutputs=1  omode=boolean  otype=uint(addrWidth)  scale=1  rndmethod=Unbiased  factor=1  satmethod=Symmetric  shift_vec=[0 1 2 -1]  value=0  inPortNames=['+'; '+';]  outPortNames=[' ']  image=dspba_prim.jpg  text=fprintf('%s', num2str(value));  style=Optimised  visibilities=8 + 1024  version=20090407
  Mux1 : DSPBAPrim/Mux  primtype=mux  nInputs=evalAionMaskParam(gcb,'value',1)+1  nOutputs=1  omode=Inherit via internal rule  otype=sfix(16)  scale=2^-15  rndmethod=Unbiased  factor=1  satmethod=Symmetric  shift_vec=[0 1 2 -1]  value=2  inPortNames=['s'; 'd0'; 'd1'; 'd2'; 'd3'; 'd4'; 'd5'; 'd6'; 'd7'; 'd8'; 'd9';]  outPortNames=[' ']  image=dspba_prim.jpg  text=fprintf('%s', primtype);  style=Optimised  visibilities=1032  version=20090623
  out_valid : Outport
  wires:
  Const8/1 -> CmpNE/2
  CmpNE/1 -> Mux1/1
  Const9/1 -> Mux1/3
  in_valid/1 -> Mux1/2
  Mux1/1 -> out_valid/1
  coeff_cnt/1 -> CmpNE/1

== system vardownsampler/FilterSystem/gen_addr_control/mem_cnt ==
  transig : Inport
  rate : Inport  Port=2
  AddSLoad1 : DSPBAPrim/AddSLoad  primtype=addsload  nInputs=4  nOutputs=1  omode=Specify via dialog  otype=uint(memAddrWidth)  scale=1  rndmethod=Unbiased  factor=1  satmethod=Symmetric  shift_vec=[0 1 2 -1]  value=0  inPortNames=['+'; '+'; 's'; 'v']  outPortNames=[' ']  image=dspba_prim.jpg  text=fprintf('+');  style=Optimised  visibilities=8  version=20090407
  CmpEQ1 : DSPBAPrim/CmpEQ  primtype=cmpeq  nInputs=2  nOutputs=1  omode=boolean  otype=sfix(16)  scale=2^-15  rndmethod=Unbiased  factor=1  satmethod=Symmetric  shift_vec=[0 1 2 -1]  value=0  inPortNames=[' '; ' ';]  outPortNames=[' ']  image=dspba_prim.jpg  text=fprintf('==');  style=Optimised  visibilities=0  version=20090407
  Const4 : DSPBAPrim/Const  primtype=const  nInputs=0  nOutputs=1  omode=Specify via dialog  otype=uint(memAddrWidth)  scale=1  rndmethod=Unbiased  factor=1  satmethod=Symmetric  shift_vec=[0 1 2 -1]  value=1  inPortNames=['+'; '+';]  outPortNames=[' ']  image=dspba_prim.jpg  text=fprintf('%s', num2str(value));  style=Optimised  visibilities=8 + 1024  version=20090407
  Const5 : DSPBAPrim/Const  primtype=const  nInputs=0  nOutputs=1  omode=Specify via dialog  otype=uint(memAddrWidth)  scale=1  rndmethod=Unbiased  factor=1  satmethod=Symmetric  shift_vec=[0 1 2 -1]  value=Period  inPortNames=['+'; '+';]  outPortNames=[' ']  image=dspba_prim.jpg  text=fprintf('%s', num2str(value));  style=Optimised  visibilities=8 + 1024  version=20090407
  Const6 : DSPBAPrim/Const  primtype=const  nInputs=0  nOutputs=1  omode=Specify via dialog  otype=uint(memAddrWidth)  scale=1  rndmethod=Unbiased  factor=1  satmethod=Symmetric  shift_vec=[0 1 2 -1]  value=1  inPortNames=['+'; '+';]  outPortNames=[' ']  image=dspba_prim.jpg  text=fprintf('%s', num2str(value));  style=Optimised  visibilities=8 + 1024  version=20090407
  Const7 : DSPBAPrim/Const  primtype=const  nInputs=0  nOutputs=1  omode=Specify via dialog  otype=uint(memAddrWidth)  scale=1  rndmethod=Unbiased  factor=1  satmethod=Symmetric  shift_vec=[0 1 2 -1]  value=0  inPortNames=['+'; '+';]  outPortNames=[' ']  image=dspba_prim.jpg  text=fprintf('%s', num2str(value));  style=Optimised  visibilities=8 + 1024  version=20090407
  Convert : DSPBAPrim/Convert  primtype=convert  nInputs=1  nOutputs=1  omode=Specify via dialog  otype=uint(memAddrWidth)  scale=1  rndmethod=Truncate  factor=1  satmethod=None  shift_vec=[0 1 2 -1]  value=round([0:255]/17)  inPortNames=[' '; ' ';]  outPortNames=[' '; 'c']  image=dspba_prim.jpg  text=fprintf('convert');  style=Optimised  visibilities=8+64+256  clipdetect=off  version=20090611
  Mult : DSPBAPrim/Mult  primtype=mult  nInputs=2  nOutputs=1  omode=Inherit via internal rule  otype=sfix(16)  scale=2^-15  rndmethod=Unbiased  factor=1  satmethod=Symmetric  shift_vec=[0 1 2 -1]  value=0  inPortNames=[' '; ' ';]  outPortNames=[' ']  image=dspba_prim.jpg  text=fprintf('X');  style=Optimised  visibilities=8  version=20090407
  Or : DSPBAPrim/Or  primtype=or  nInputs=2  nOutputs=1  omode=Inherit via internal rule  otype=sfix(16)  scale=2^-15  rndmethod=Unbiased  factor=1  satmethod=Symmetric  shift_vec=[0 1 2 -1]  value=0  inPortNames=[' '; ' '; ' '; ' '; ' '; ' '; ' '; ' '; ' '; ' '; ' '; ' '; ' '; ' '; ' '; ' '; ]  outPortNames=[' ']  image=dspba_prim.jpg  text=fprintf('|');  style=Optimised  visibilities=8+2  version=20090407
  SampleDelay1 : DSPBAPrim/SampleDelay  primtype=sampdelay  nInputs=1  nOutputs=1  omode=Specify via dialog  otype=uint(memAddrWidth)  scale=1  rndmethod=Unbiased  factor=1  satmethod=Symmetric  shift_vec=[0 1 2 -1]  value=1  inPortNames=[' '; ' ';]  outPortNames=[' ']  image=dspba_prim.jpg  text=dpoly(1, eye(1,value+1), 'z')  style=Optimised  visibilities=8 + 1024  version=20090407
  Sub1 : DSPBAPrim/Sub  primtype=sub  nInputs=2  nOutputs=1  omode=Specify via dialog  otype=uint(memAddrWidth)  scale=1  rndmethod=Unbiased  factor=1  satmethod=Symmetric  shift_vec=[0 1 2 -1]  value=0  inPortNames=['+'; '-';]  outPortNames=[' ']  image=dspba_prim.jpg  text=fprintf('-');  style=Optimised  visibilities=8  version=20090407
  mem_cnt : Outport
  wires:
  Const4/1 -> Sub1/2
  Mult/1 -> Convert/1
  Sub1/1 -> CmpEQ1/2
  Const5/1 -> Mult/2
  Const6/1 -> AddSLoad1/2
  AddSLoad1/1 -> SampleDelay1/1, mem_cnt/1
  Const7/1 -> AddSLoad1/4
  rate/1 -> Mult/1
  Convert/1 -> Sub1/1
  transig/1 -> Or/1
  Or/1 -> AddSLoad1/3
  CmpEQ1/1 -> Or/2
  SampleDelay1/1 -> AddSLoad1/1, CmpEQ1/1
